simulink model "TP24_A47521"  (R2018b)
settings: Solver=ode15s  StartTime=0.0  StopTime=0.2  RelTol=1e-3
settings Model: SnapshotInterval=1  Creator=joaov  LastModifiedBy=A47521
settings DataIOCC: ReturnWorkspaceOutputs=on

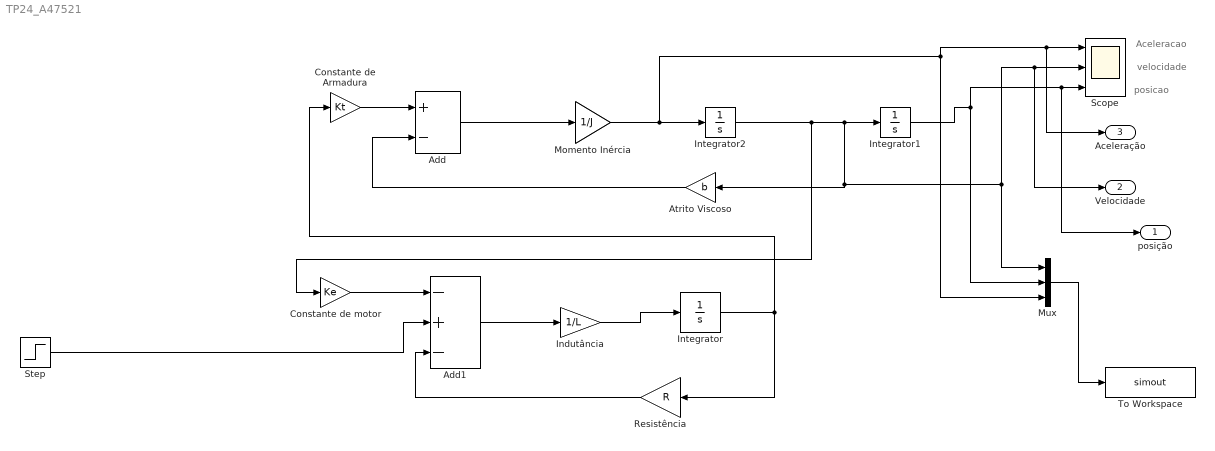
== system TP24_A47521 ==
  note: posicao
  note: velocidade
  note: Aceleracao
  Add : Sum  Inputs=+-
  Add1 : Sum  Inputs=-+-
  Atrito Viscoso : Gain  Gain=b  mask{b=0.000003}
      mask prompts: b "Atrito Viscoso"
  Constante de Armadura : Gain  Gain=Kt  mask{Kt=0.02}
      mask prompts: Kt "Constante de Armadura"
  Constante de motor : Gain  Gain=Ke  mask{Ke=0.02}
      mask prompts: Ke "Constante de Motor"
  Indutância : Gain  Gain=1/L  mask{L=0.0000027}
      mask prompts: L "Indutância"
  Integrator : Integrator
  Integrator1 : Integrator
  Integrator2 : Integrator
  Momento Inércia : Gain  Gain=1/J  mask{J=0.0000032}
      mask prompts: J "Momento de Inércia"
  Mux : Mux  Inputs=3
  Resistência : Gain  Gain=R  mask{R=4}
      mask prompts: R "Resistência Elétrica"
  Scope : Scope  NumInputPorts=3
  Step : Step  Time=0  SampleTime=0
  To Workspace : ToWorkspace  VariableName=simout  SaveFormat=Timeseries  SampleTime=-1
  posição : Outport  VectorParamsAs1DForOutWhenUnconnected=on
  Velocidade : Outport  Port=2  VectorParamsAs1DForOutWhenUnconnected=on
  Aceleração : Outport  Port=3  VectorParamsAs1DForOutWhenUnconnected=on
  wires:
  Add1/1 -> Indutância/1
  Add/1 -> Momento Inércia/1
  Step/1 -> Add1/2
  Indutância/1 -> Integrator/1
  Resistência/1 -> Add1/3
  Constante de Armadura/1 -> Add/1
  Integrator/1 -> Resistência/1, Constante de Armadura/1
  Momento Inércia/1 -> Aceleração/1, Scope/1, Mux/3, Integrator2/1
  Atrito Viscoso/1 -> Add/2
  Constante de motor/1 -> Add1/1
  Integrator2/1 -> Velocidade/1, Scope/2, Mux/1, Atrito Viscoso/1, Integrator1/1, Constante de motor/1
  Integrator1/1 -> Mux/2, posição/1, Scope/3
  Mux/1 -> To Workspace/1
